simulink model "SP_sim_using_MATLAB_Function"  (R2021b)
settings: Solver=VariableStepAuto  StartTime=0.0  StopTime=10.0  RelTol=1e-3
values from neighbouring files (symbols this model uses):
  g = 9.80665    [SP_Parameters.m]
  k = 0.2    [SP_Parameters.m]
  l = 1.5    [SP_Parameters.m]
  S0 = [pi/4 ,2]    [SP_Parameters.m]
settings Model: Creator=Sushmanth Sai G  LastModifiedBy=Sushmanth Sai G

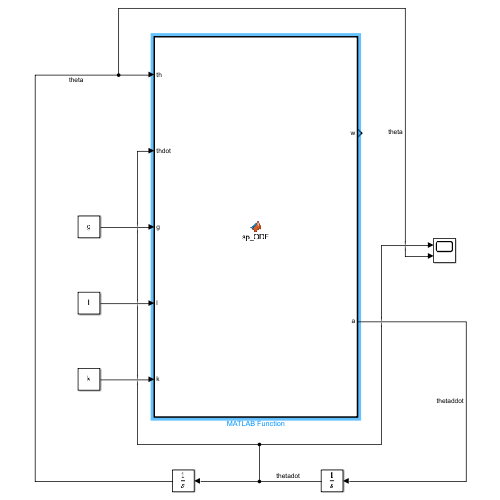
[thumbnail: Simulink's stored preview of the top-level diagram]
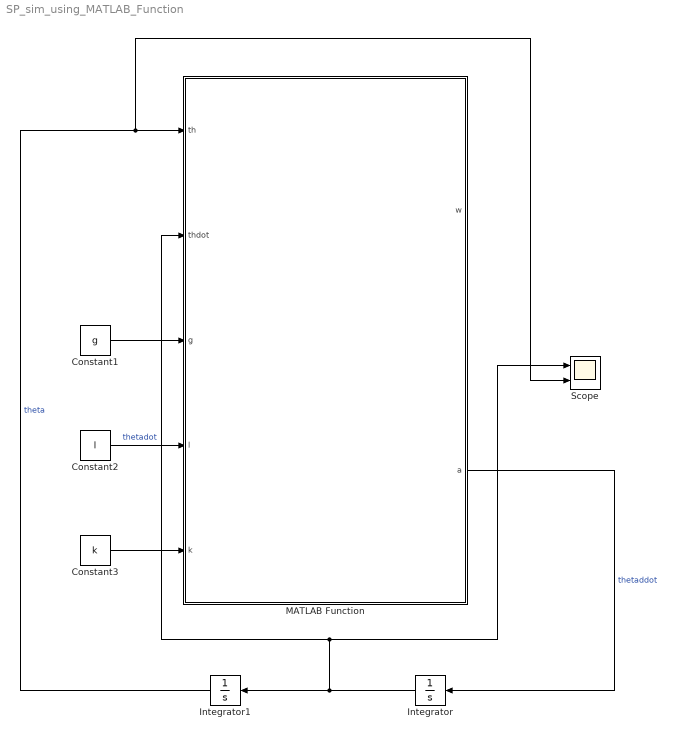
== system SP_sim_using_MATLAB_Function ==
  Constant1 : Constant  Value=g
  Constant2 : Constant  Value=l
  Constant3 : Constant  Value=k
  Integrator : Integrator  InitialCondition=S0(2)
  Integrator1 : Integrator  InitialCondition=S0(1)
  MATLAB Function : MATLAB Function  TreatAsAtomicUnit=on
  Scope : Scope  NumInputPorts=2
  wires:
  Constant1/1 -> MATLAB Function/3(g)
  Constant2/1 -> MATLAB Function/4(l)
  Constant3/1 -> MATLAB Function/5(k)
  MATLAB Function/2(a) -> Integrator/1  "thetaddot"
  Integrator/1 -> Scope/1, MATLAB Function/2(thdot), Integrator1/1  "thetadot"
  Integrator1/1 -> Scope/2, MATLAB Function/1(th)  "theta"

== matlab function SP_sim_using_MATLAB_Function/MATLAB Function ==
  data: th input; thdot input; g input; w output; l input; a output; k input

function [w,a] = sp_ODE(th,thdot,g,l,k)

w = thdot;
a = -(g/l)*sin(th - 3*pi/2) - k*thdot;

end
